simulink model "symulink"  (R2021b)
settings: Solver=VariableStepAuto  StartTime=0.0  StopTime=20.0  RelTol=1e-3
undefined symbols (not defined in the file): Hf, R
settings Model: Creator=pacur  LastModifiedBy=pacur

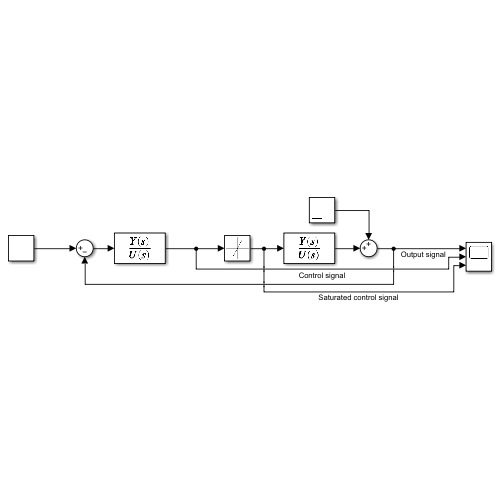
[thumbnail: Simulink's stored preview of the top-level diagram]
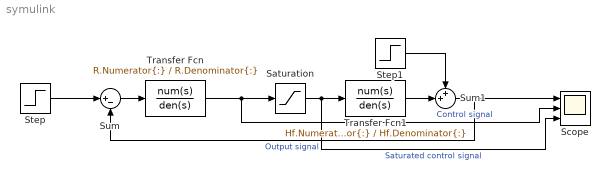
== system symulink ==
  Saturation : Saturate  UpperLimit=1  LowerLimit=-1
  Scope : Scope  NumInputPorts=3
  Step : Step  SampleTime=0
  Step1 : Step  Time=10  After=5  SampleTime=0
  Sum : Sum  Inputs=|+-
  Sum1 : Sum  Inputs=++|
  Transfer Fcn : TransferFcn  Numerator=R.Numerator{:}  Denominator=R.Denominator{:}
  Transfer Fcn1 : TransferFcn  Numerator=Hf.Numerator{:}  Denominator=Hf.Denominator{:}
  wires:
  Step/1 -> Sum/1
  Sum/1 -> Transfer Fcn/1
  Saturation/1 -> Scope/3, Transfer Fcn1/1  "Saturated control signal"
  Transfer Fcn1/1 -> Sum1/2
  Step1/1 -> Sum1/1
  Sum1/1 -> Scope/1, Sum/2  "Output signal"
  Transfer Fcn/1 -> Scope/2, Saturation/1  "Control signal"
